simulink model "simulink_simulation"  (R2018b)
settings: Solver=VariableStepAuto  StartTime=0.0  StopTime=10.0  RelTol=1e-3
libraries: simulink x2
settings Model: Creator=Mahban  LastModifiedBy=Mahban
settings DataIOCC: ReturnWorkspaceOutputs=on
settings DebuggingCC: SFMachineParentedDataDiag=error

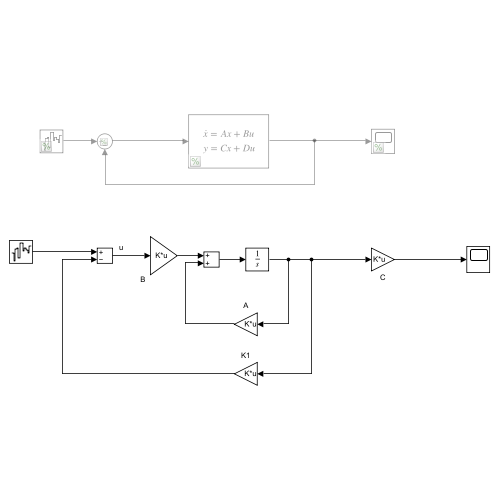
[thumbnail: Simulink's stored preview of the top-level diagram]
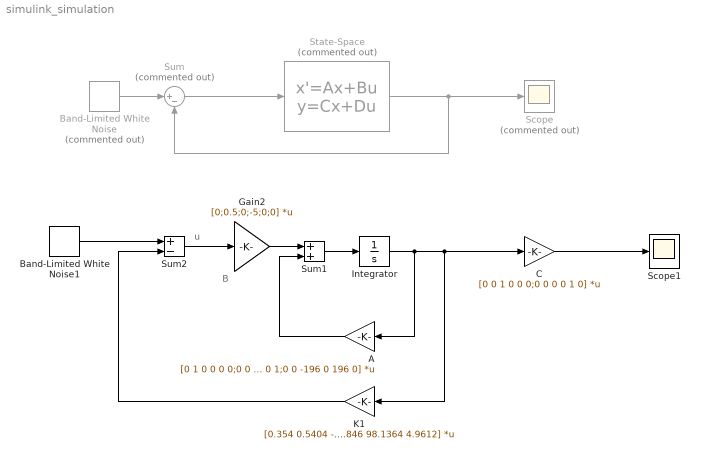
== system simulink_simulation ==
  note: u
  note: B
  A : Gain  Gain=[0 1 0 0 0 0;0 0 -0.98 0 0 0;0 0 0 1 0 0;0 0 205.8 0 -98 0;0 0 0 0 0 1;0 0 -196 0 196 0]  Multiplication=Matrix(K*u)
  Band-Limited White Noise : simulink/Sources/Band-Limited White Noise  Commented=on  Cov=[0.1]  Ts=0.1  seed=[23341]
  Band-Limited White Noise1 : simulink/Sources/Band-Limited White Noise  Cov=[0.1]  Ts=0.1  seed=[23341]
  C : Gain  Gain=[0 0 1 0 0 0;0 0 0 0 1 0]  Multiplication=Matrix(K*u)
  Gain2 : Gain  Gain=[0;0.5;0;-5;0;0]  Multiplication=Matrix(K*u)
  Integrator : Integrator  InitialCondition=zeros(6,1)
  K1 : Gain  Gain=[0.354 0.5404 -116.4246 -3.846 98.1364 4.9612]  Multiplication=Matrix(K*u)
  Scope : Scope  Commented=on
  Scope1 : Scope
  State-Space : StateSpace  Commented=on  A=[0 1 0 0 0 0;0 0 -0.98 0 0 0;0 0 0 1 0 0;0 0 205.8 0 -98 0;0 0 0 0 0 1;0 0 -196 0 196 0]  B=[0;0.5;0;-5;0;0]  C=[0 0 1 0 0 0;0 0 0 0 1 0]  D=[0;0]  InitialCondition=0
  Sum : Sum  Commented=on  Inputs=|+-
  Sum1 : Sum
  Sum2 : Sum  Inputs=+-
  wires:
  Band-Limited White Noise/1 -> Sum/1
  Sum/1 -> State-Space/1
  State-Space/1 -> Scope/1, Sum/2
  Band-Limited White Noise1/1 -> Sum2/1
  A/1 -> Sum1/2
  Integrator/1 -> A/1, C/1, K1/1
  Sum2/1 -> Gain2/1
  Sum1/1 -> Integrator/1
  K1/1 -> Sum2/2
  Gain2/1 -> Sum1/1
  C/1 -> Scope1/1
